simulink model "SchemaControlloDecentralizzatoSmartSixR2013a"  (Simulink 8.4)
settings: Solver=ode23  StartTime=0.0  StopTime=t(end)+Tf  FixedStep=T  RelTol=1e-3
PreLoadFcn:
  | initFunction
InitFcn:
  | initFunction
StopFcn:
  | figure
  | subplot(31,1)
  | plot(err_q.data(1:50))
  | subplot(312)
  | plot(err_dq.data(1:50))
  | subplot(313)
  | plot(err_ddq.data(1:50))
values from neighbouring files (symbols this model uses):
  FM = Kr^-1*Fv*Kr^-1    [ControlloreUnico.m]    (also in SimulazioneLsim.m = Kr^-1*Fv_att*Kr^-1; initFunction.m; initFunctionIm.m)
  Im = Kr^-1*Bconst*Kr^-1    [initFunction.m]    (also in initFunctionIm.m)
  KCA = diag([(-W(1,1)^2 + KM(1,1)*XR(1,1))/(KM(1,1)*KTA(1,1)*W(1,1)^2),             (-W(2,2)^2 + KM(2,2)*XR(2,2))/(KM(2,2)*KTA(2,2)*W(2,2)^2),             (-W(3,3)^2 + KM(3,3)*XR(3,3))/(KM(3,3)*KTA(3,3)*W(3,3)^2),             (-W(4,4)^2 + KM(4,4)*XR(4,4))/(KM(4,4)*KTA(4,4)*W(4,4)^2),             (-W(5,5)^2 + KM(5,5)*XR(5,5))/(KM(5,5)*KTA(5,5)*W(5,5)^2),             (-W(6,6)^2 + KM(6,6)*XR(6,6))/(KM(6,6)* ...(+20 chars)    [DesignControllersAcceleration_6.m]    (also in DesignControllersAcceleration_7.m; DiscreteControllersAcceleration_7.m)
  KCP = diag([(KTV(1,1)*W(1,1))/(2*KTP(1,1)*Z(1,1)),             (KTV(2,2)*W(2,2))/(2*KTP(2,2)*Z(2,2)),             (KTV(3,3)*W(3,3))/(2*KTP(3,3)*Z(3,3)),             (KTV(4,4)*W(4,4))/(2*KTP(4,4)*Z(4,4)),             (KTV(5,5)*W(5,5))/(2*KTP(5,5)*Z(5,5)),             (KTV(6,6)*W(6,6))/(2*KTP(6,6)*Z(6,6))])    [DesignControllersAcceleration_6.m]    (also in DesignControllersAcceleration_7.m; DesignControllersVelocity_6.m; DiscreteControllersAcceleration_7.m; DiscreteDesignControllersVelocity_6.m)
  KCV = diag([(2*KM(1,1)*KTA(1,1)*W(1,1)*XR(1,1)*Z(1,1))/(KTV(1,1)*(-W(1,1)^2 + KM(1,1)*XR(1,1))),             (2*KM(2,2)*KTA(2,2)*W(2,2)*XR(2,2)*Z(2,2))/(KTV(2,2)*(-W(2,2)^2 + KM(2,2)*XR(2,2))),             (2*KM(3,3)*KTA(3,3)*W(3,3)*XR(3,3)*Z(3,3))/(KTV(3,3)*(-W(3,3)^2 + KM(3,3)*XR(3,3))),             (2*KM(4,4)*KTA(4,4)*W(4,4)*XR(4,4)*Z(4,4))/(KTV(4,4)*(-W(4,4)^2 + KM(4,4)*XR(4,4))),             (2*KM( ...(+176 chars)    [DesignControllersAcceleration_6.m]    (also in DesignControllersAcceleration_7.m; DesignControllersVelocity_6.m = diag([(2*W(1,1)*Z(1,1))/(KM(1,1)*KTV(1,1)),             (2*W; DiscreteControllersAcceleration_7.m = diag([(rlkcv(1)*KM(1,1)*KTA(1,1)*W(1,1)*XR(1,1)*Z(1,1))/(KTV; DiscreteDesignControllersVelocity_6.m = diag([rlkcv(1)*(2*W(1,1)*Z(1,1))/(KM(1,1)*KTV(1,1)),        )
  KM = Kv^-1    [DesignControllersAcceleration_6.m]    (also in DesignControllersAcceleration_7.m; DesignControllersVelocity_6.m; DiscreteControllersAcceleration_7.m; DiscreteDesignControllersVelocity_6.m)
  KTA = diag([100 1 1 1 1 1])    [DesignControllersAcceleration_6.m]    (also in DesignControllersAcceleration_7.m = diag([1 1 1 1 1 1]); DiscreteControllersAcceleration_7.m = diag([1 1 1 1 1 1]))
  KTP = diag([9 1 1 1 1 1])    [DesignControllersAcceleration_6.m]    (also in DesignControllersAcceleration_7.m = diag([1 1 1 1 1 1]); DesignControllersVelocity_6.m = diag([1 1 1 1 1 1]); DiscreteControllersAcceleration_7.m = diag([1 1 1 1 1 1]); DiscreteDesignControllersVelocity_6.m = diag([1 1 1 1 1 1]))
  KTV = diag([4 1 1 1 1 1])    [DesignControllersAcceleration_6.m]    (also in DesignControllersAcceleration_7.m = diag([1 1 1 1 1 1]); DesignControllersVelocity_6.m = diag([1 1 1 1 1 1]); DiscreteControllersAcceleration_7.m = diag([1 1 1 1 1 1]); DiscreteDesignControllersVelocity_6.m = diag([1 1 1 1 1 1]))
  q0 = q0'    [initFunction.m]    (also in initFunctionIm.m)
  T = 0.05    [ComputeBconst_4.m]    (also in ControlloreUnico.m = 0.002; Identificazione_2.m = 0:1/F:(size(min_value,2)-1)*interval; Simulazione.m = 0.002; SimulazioneLsim.m = 0.002)
  TCA = diag([Tm(1,1) Tm(2,2) Tm(3,3) Tm(4,4) Tm(5,5) Tm(6,6)])    [DesignControllersAcceleration_6.m]    (also in DesignControllersAcceleration_7.m = diag([TM(1,1) TM(2,2) TM(3,3) TM(4,4) TM(5,5) TM(6,6)]); DiscreteControllersAcceleration_7.m = diag([TM(1,1) TM(2,2) TM(3,3) TM(4,4) TM(5,5) TM(6,6)]))
undefined symbols (not defined in the file or in its folder): Kr, Kt, Kv, La, Ra
libraries: simulink x18
(part 2 of 2)

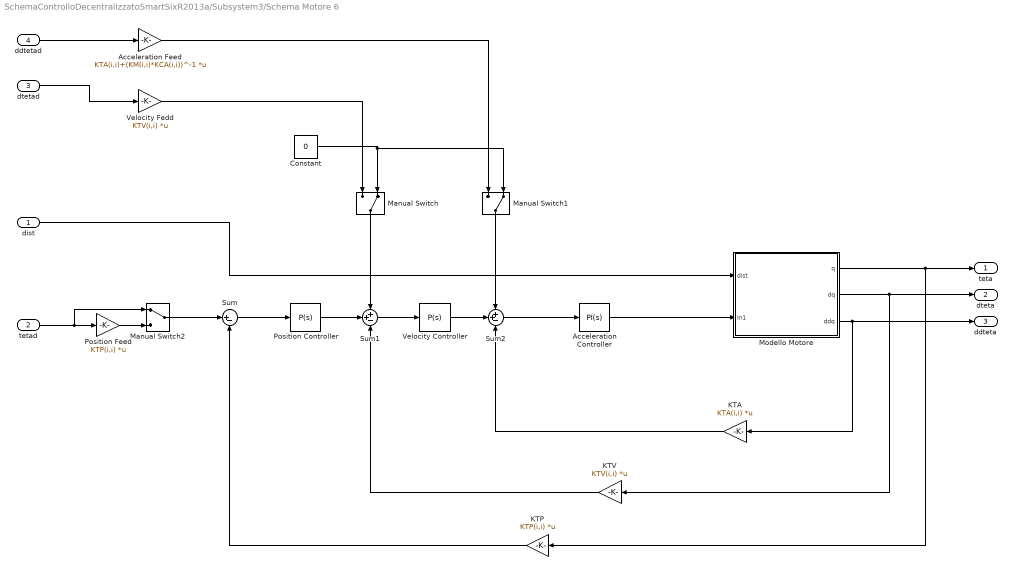
== system SchemaControlloDecentralizzatoSmartSixR2013a/Subsystem3/Schema Motore 6 ==
  dist : Inport  PortDimensions=1
  tetad : Inport  Port=2  PortDimensions=1
  dtetad : Inport  Port=3  PortDimensions=1
  ddtetad : Inport  Port=4  PortDimensions=1
  Acceleration Controller : simulink/Continuous/PID Controller  Controller=PI  TimeDomain=Continuous-time  SampleTime=-1  IntegratorMethod=Forward Euler  FilterMethod=Forward Euler  Form=Parallel  P=TCA(i,i)*KCA(i,i)  I=KCA(i,i)  D=0  N=100  InitialConditionSource=internal  InitialConditionForIntegrator=0  InitialConditionForFilter=0  ExternalReset=none  LimitOutput=off  UpperSaturationLimit=inf  LowerSaturationLimit=-inf  LinearizeAsGain=on  AntiWindupMode=none  Kb=1  TrackingMode=off  Kt=1  PParamMin=[]  PParamMax=[]  IParamMin=[]  IParamMax=[]  DParamMin=[]  DParamMax=[]  NParamMin=[]  NParamMax=[]  KbParamMin=[]  KbParamMax=[]  KtParamMin=[]  KtParamMax=[]  POutMin=[]  POutMax=[]  IOutMin=[]  IOutMax=[]  DOutMin=[]  DOutMax=[]  NOutMin=[]  NOutMax=[]  KbOutMin=[]  KbOutMax=[]  KtOutMin=[]  KtOutMax=[]  IntegratorOutMin=[]  IntegratorOutMax=[]  FilterOutMin=[]  FilterOutMax=[]  SumOutMin=[]  SumOutMax=[]  SumI1OutMin=[]  SumI1OutMax=[]  SumI2OutMin=[]  SumI2OutMax=[]  SumI3OutMin=[]  SumI3OutMax=[]  SumDOutMin=[]  SumDOutMax=[]  SaturationOutMin=[]  SaturationOutMax=[]  IntegratorContinuousStateAttributes=''  IntegratorStateMustResolveToSignalObject=off  IntegratorRTWStateStorageClass=Auto  FilterContinuousStateAttributes=''  FilterStateMustResolveToSignalObject=off  FilterRTWStateStorageClass=Auto  DifferentiatorICPrevScaledInput=0  DifferentiatorOutMin=[]  DifferentiatorOutMax=[]  UseFilter=on
  Acceleration Feed : Gain  Gain=KTA(i,i)+(KM(i,i)*KCA(i,i))^-1  Multiplication=Matrix(K*u)
  Constant : Constant  Value=0
  KTA : Gain  Gain=KTA(i,i)  Multiplication=Matrix(K*u)
  KTP : Gain  Gain=KTP(i,i)  Multiplication=Matrix(K*u)
  KTV : Gain  Gain=KTV(i,i)  Multiplication=Matrix(K*u)
  Manual Switch : ManualSwitch  CurrentSetting=0
  Manual Switch1 : ManualSwitch  CurrentSetting=0
  Manual Switch2 : ManualSwitch
  Modello Motore : Subsystem
  Position Controller : simulink/Continuous/PID Controller  Controller=P  TimeDomain=Continuous-time  SampleTime=-1  IntegratorMethod=Forward Euler  FilterMethod=Forward Euler  Form=Parallel  P=KCP(i,i)  I=1  D=0  N=100  InitialConditionSource=internal  InitialConditionForIntegrator=0  InitialConditionForFilter=0  ExternalReset=none  LimitOutput=off  UpperSaturationLimit=inf  LowerSaturationLimit=-inf  LinearizeAsGain=on  AntiWindupMode=none  Kb=1  TrackingMode=off  Kt=1  PParamMin=[]  PParamMax=[]  IParamMin=[]  IParamMax=[]  DParamMin=[]  DParamMax=[]  NParamMin=[]  NParamMax=[]  KbParamMin=[]  KbParamMax=[]  KtParamMin=[]  KtParamMax=[]  POutMin=[]  POutMax=[]  IOutMin=[]  IOutMax=[]  DOutMin=[]  DOutMax=[]  NOutMin=[]  NOutMax=[]  KbOutMin=[]  KbOutMax=[]  KtOutMin=[]  KtOutMax=[]  IntegratorOutMin=[]  IntegratorOutMax=[]  FilterOutMin=[]  FilterOutMax=[]  SumOutMin=[]  SumOutMax=[]  SumI1OutMin=[]  SumI1OutMax=[]  SumI2OutMin=[]  SumI2OutMax=[]  SumI3OutMin=[]  SumI3OutMax=[]  SumDOutMin=[]  SumDOutMax=[]  SaturationOutMin=[]  SaturationOutMax=[]  IntegratorContinuousStateAttributes=''  IntegratorStateMustResolveToSignalObject=off  IntegratorRTWStateStorageClass=Auto  FilterContinuousStateAttributes=''  FilterStateMustResolveToSignalObject=off  FilterRTWStateStorageClass=Auto  DifferentiatorICPrevScaledInput=0  DifferentiatorOutMin=[]  DifferentiatorOutMax=[]  UseFilter=on
  Position Feed : Gain  Gain=KTP(i,i)  Multiplication=Matrix(K*u)
  Sum : Sum  Inputs=|+-
  Sum1 : Sum  Inputs=++-
  Sum2 : Sum  Inputs=++-
  Velocity Controller : simulink/Continuous/PID Controller  Controller=P  TimeDomain=Continuous-time  SampleTime=-1  IntegratorMethod=Forward Euler  FilterMethod=Forward Euler  Form=Parallel  P=KCV(i,i)  I=1  D=0  N=100  InitialConditionSource=internal  InitialConditionForIntegrator=0  InitialConditionForFilter=0  ExternalReset=none  LimitOutput=off  UpperSaturationLimit=inf  LowerSaturationLimit=-inf  LinearizeAsGain=on  AntiWindupMode=none  Kb=1  TrackingMode=off  Kt=1  PParamMin=[]  PParamMax=[]  IParamMin=[]  IParamMax=[]  DParamMin=[]  DParamMax=[]  NParamMin=[]  NParamMax=[]  KbParamMin=[]  KbParamMax=[]  KtParamMin=[]  KtParamMax=[]  POutMin=[]  POutMax=[]  IOutMin=[]  IOutMax=[]  DOutMin=[]  DOutMax=[]  NOutMin=[]  NOutMax=[]  KbOutMin=[]  KbOutMax=[]  KtOutMin=[]  KtOutMax=[]  IntegratorOutMin=[]  IntegratorOutMax=[]  FilterOutMin=[]  FilterOutMax=[]  SumOutMin=[]  SumOutMax=[]  SumI1OutMin=[]  SumI1OutMax=[]  SumI2OutMin=[]  SumI2OutMax=[]  SumI3OutMin=[]  SumI3OutMax=[]  SumDOutMin=[]  SumDOutMax=[]  SaturationOutMin=[]  SaturationOutMax=[]  IntegratorContinuousStateAttributes=''  IntegratorStateMustResolveToSignalObject=off  IntegratorRTWStateStorageClass=Auto  FilterContinuousStateAttributes=''  FilterStateMustResolveToSignalObject=off  FilterRTWStateStorageClass=Auto  DifferentiatorICPrevScaledInput=0  DifferentiatorOutMin=[]  DifferentiatorOutMax=[]  UseFilter=on
  Velocity Fedd : Gain  Gain=KTV(i,i)  Multiplication=Matrix(K*u)
  teta : Outport  PortDimensions=1
  dteta : Outport  Port=2  PortDimensions=1
  ddteta : Outport  Port=3  PortDimensions=1
  wires:
  Sum/1 -> Position Controller/1
  Sum1/1 -> Velocity Controller/1
  Sum2/1 -> Acceleration Controller/1
  ddtetad/1 -> Acceleration Feed/1
  KTP/1 -> Sum/2
  Acceleration Controller/1 -> Modello Motore/2(In1)
  dist/1 -> Modello Motore/1(dist)
  Modello Motore/2(dq) -> dteta/1, KTV/1
  Modello Motore/1(q) -> teta/1, KTP/1
  Modello Motore/3(ddq) -> ddteta/1, KTA/1
  Position Controller/1 -> Sum1/2
  KTV/1 -> Sum1/3
  Manual Switch/1 -> Sum1/1
  KTA/1 -> Sum2/3
  Velocity Controller/1 -> Sum2/2
  Constant/1 -> Manual Switch1/2, Manual Switch/2
  Manual Switch1/1 -> Sum2/1
  tetad/1 -> Position Feed/1, Manual Switch2/1
  Manual Switch2/1 -> Sum/1
  Position Feed/1 -> Manual Switch2/2
  Velocity Fedd/1 -> Manual Switch/1
  Acceleration Feed/1 -> Manual Switch1/1
  dtetad/1 -> Velocity Fedd/1

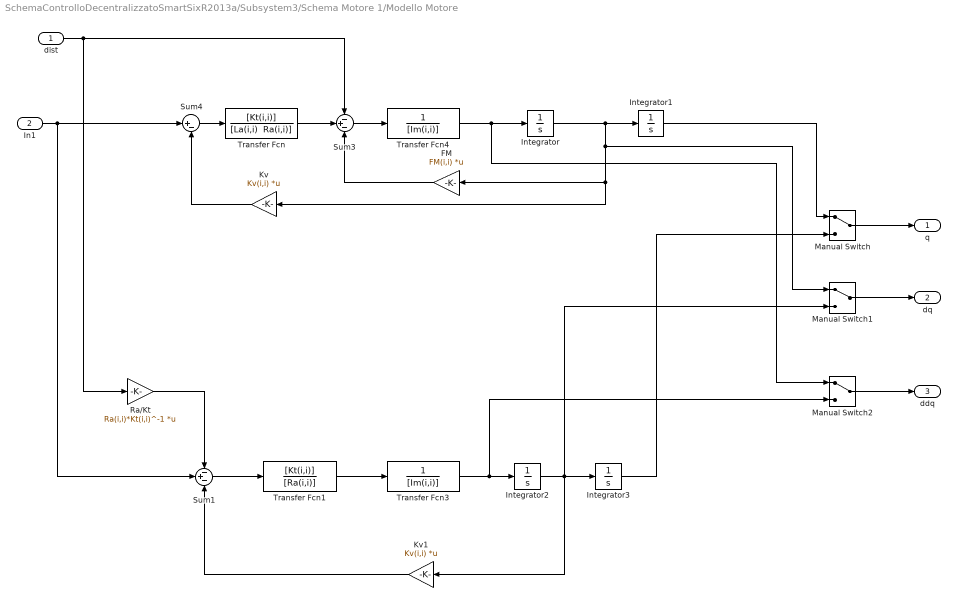
== system SchemaControlloDecentralizzatoSmartSixR2013a/Subsystem3/Schema Motore 1/Modello Motore ==
  dist : Inport
  In1 : Inport  Port=2
  FM : Gain  Gain=FM(i,i)  Multiplication=Matrix(K*u)
  Integrator : Integrator
  Integrator1 : Integrator  InitialCondition=q0(i)
  Integrator2 : Integrator
  Integrator3 : Integrator  InitialCondition=q0(i)
  Kv : Gain  Gain=Kv(i,i)  Multiplication=Matrix(K*u)
  Kv1 : Gain  Gain=Kv(i,i)  Multiplication=Matrix(K*u)
  Manual Switch : ManualSwitch
  Manual Switch1 : ManualSwitch
  Manual Switch2 : ManualSwitch
  Ra/Kt : Gain  Gain=Ra(i,i)*Kt(i,i)^-1  Multiplication=Matrix(K*u)
  Sum1 : Sum  Inputs=-+-
  Sum3 : Sum  Inputs=-+-
  Sum4 : Sum  Inputs=|+-
  Transfer Fcn : TransferFcn  Numerator=[Kt(i,i)]  Denominator="[La(i,i)  Ra(i,i)]"
  Transfer Fcn1 : TransferFcn  Numerator=[Kt(i,i)]  Denominator=[Ra(i,i)]
  Transfer Fcn3 : TransferFcn  Denominator=[Im(i,i)]
  Transfer Fcn4 : TransferFcn  Denominator=[Im(i,i)]
  q : Outport
  dq : Outport  Port=2
  ddq : Outport  Port=3
  wires:
  Manual Switch2/1 -> ddq/1
  Manual Switch1/1 -> dq/1
  Manual Switch/1 -> q/1
  Integrator/1 -> Kv/1, FM/1, Manual Switch1/1, Integrator1/1
  Kv/1 -> Sum4/2
  In1/1 -> Sum1/2, Sum4/1
  Sum4/1 -> Transfer Fcn/1
  Transfer Fcn/1 -> Sum3/2
  FM/1 -> Sum3/3
  Integrator1/1 -> Manual Switch/1
  dist/1 -> Ra/Kt/1, Sum3/1
  Ra/Kt/1 -> Sum1/1
  Sum1/1 -> Transfer Fcn1/1
  Transfer Fcn1/1 -> Transfer Fcn3/1
  Transfer Fcn3/1 -> Manual Switch2/2, Integrator2/1
  Integrator2/1 -> Manual Switch1/2, Kv1/1, Integrator3/1
  Kv1/1 -> Sum1/3
  Integrator3/1 -> Manual Switch/2
  Sum3/1 -> Transfer Fcn4/1
  Transfer Fcn4/1 -> Manual Switch2/1, Integrator/1

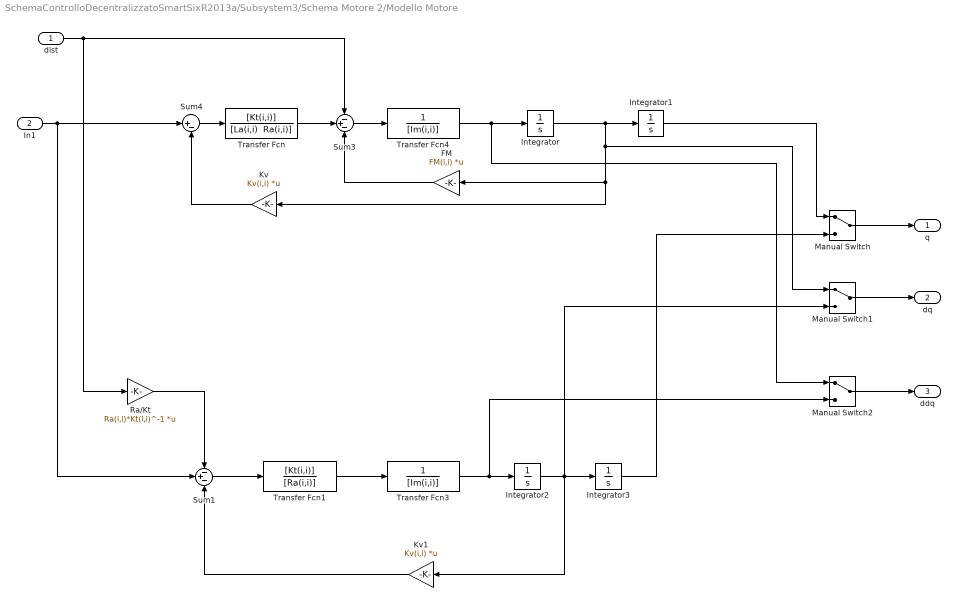
== system SchemaControlloDecentralizzatoSmartSixR2013a/Subsystem3/Schema Motore 2/Modello Motore ==
  dist : Inport
  In1 : Inport  Port=2
  FM : Gain  Gain=FM(i,i)  Multiplication=Matrix(K*u)
  Integrator : Integrator
  Integrator1 : Integrator  InitialCondition=q0(i)
  Integrator2 : Integrator
  Integrator3 : Integrator  InitialCondition=q0(i)
  Kv : Gain  Gain=Kv(i,i)  Multiplication=Matrix(K*u)
  Kv1 : Gain  Gain=Kv(i,i)  Multiplication=Matrix(K*u)
  Manual Switch : ManualSwitch
  Manual Switch1 : ManualSwitch
  Manual Switch2 : ManualSwitch
  Ra/Kt : Gain  Gain=Ra(i,i)*Kt(i,i)^-1  Multiplication=Matrix(K*u)
  Sum1 : Sum  Inputs=-+-
  Sum3 : Sum  Inputs=-+-
  Sum4 : Sum  Inputs=|+-
  Transfer Fcn : TransferFcn  Numerator=[Kt(i,i)]  Denominator="[La(i,i)  Ra(i,i)]"
  Transfer Fcn1 : TransferFcn  Numerator=[Kt(i,i)]  Denominator=[Ra(i,i)]
  Transfer Fcn3 : TransferFcn  Denominator=[Im(i,i)]
  Transfer Fcn4 : TransferFcn  Denominator=[Im(i,i)]
  q : Outport
  dq : Outport  Port=2
  ddq : Outport  Port=3
  wires:
  Manual Switch2/1 -> ddq/1
  Manual Switch1/1 -> dq/1
  Manual Switch/1 -> q/1
  Integrator/1 -> Kv/1, FM/1, Manual Switch1/1, Integrator1/1
  Kv/1 -> Sum4/2
  In1/1 -> Sum1/2, Sum4/1
  Sum4/1 -> Transfer Fcn/1
  Transfer Fcn/1 -> Sum3/2
  FM/1 -> Sum3/3
  Integrator1/1 -> Manual Switch/1
  dist/1 -> Ra/Kt/1, Sum3/1
  Ra/Kt/1 -> Sum1/1
  Sum1/1 -> Transfer Fcn1/1
  Transfer Fcn1/1 -> Transfer Fcn3/1
  Transfer Fcn3/1 -> Manual Switch2/2, Integrator2/1
  Integrator2/1 -> Manual Switch1/2, Kv1/1, Integrator3/1
  Kv1/1 -> Sum1/3
  Integrator3/1 -> Manual Switch/2
  Sum3/1 -> Transfer Fcn4/1
  Transfer Fcn4/1 -> Manual Switch2/1, Integrator/1

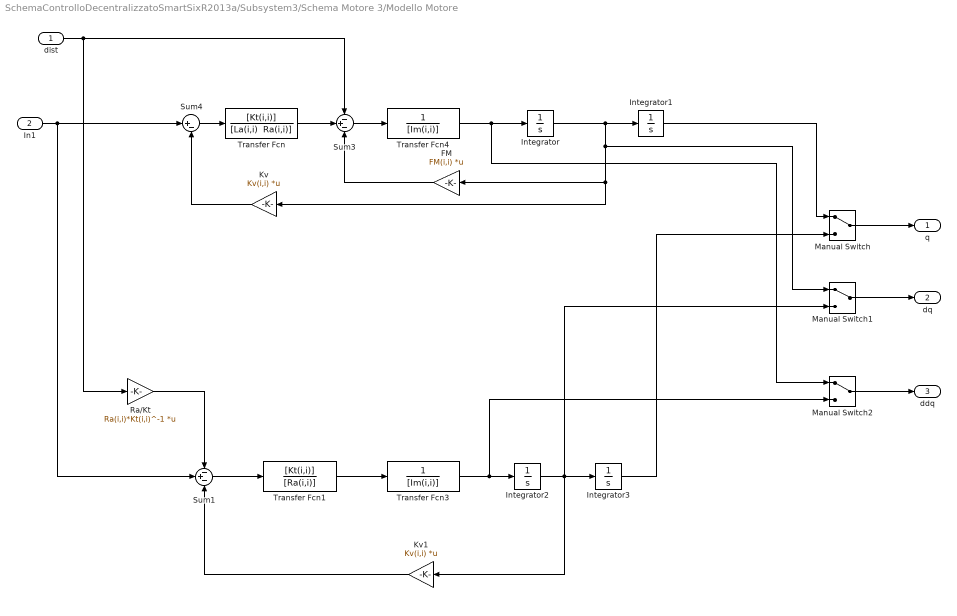
== system SchemaControlloDecentralizzatoSmartSixR2013a/Subsystem3/Schema Motore 3/Modello Motore ==
  dist : Inport
  In1 : Inport  Port=2
  FM : Gain  Gain=FM(i,i)  Multiplication=Matrix(K*u)
  Integrator : Integrator
  Integrator1 : Integrator  InitialCondition=q0(i)
  Integrator2 : Integrator
  Integrator3 : Integrator  InitialCondition=q0(i)
  Kv : Gain  Gain=Kv(i,i)  Multiplication=Matrix(K*u)
  Kv1 : Gain  Gain=Kv(i,i)  Multiplication=Matrix(K*u)
  Manual Switch : ManualSwitch
  Manual Switch1 : ManualSwitch
  Manual Switch2 : ManualSwitch
  Ra/Kt : Gain  Gain=Ra(i,i)*Kt(i,i)^-1  Multiplication=Matrix(K*u)
  Sum1 : Sum  Inputs=-+-
  Sum3 : Sum  Inputs=-+-
  Sum4 : Sum  Inputs=|+-
  Transfer Fcn : TransferFcn  Numerator=[Kt(i,i)]  Denominator="[La(i,i)  Ra(i,i)]"
  Transfer Fcn1 : TransferFcn  Numerator=[Kt(i,i)]  Denominator=[Ra(i,i)]
  Transfer Fcn3 : TransferFcn  Denominator=[Im(i,i)]
  Transfer Fcn4 : TransferFcn  Denominator=[Im(i,i)]
  q : Outport
  dq : Outport  Port=2
  ddq : Outport  Port=3
  wires:
  Manual Switch2/1 -> ddq/1
  Manual Switch1/1 -> dq/1
  Manual Switch/1 -> q/1
  Integrator/1 -> Kv/1, FM/1, Manual Switch1/1, Integrator1/1
  Kv/1 -> Sum4/2
  In1/1 -> Sum1/2, Sum4/1
  Sum4/1 -> Transfer Fcn/1
  Transfer Fcn/1 -> Sum3/2
  FM/1 -> Sum3/3
  Integrator1/1 -> Manual Switch/1
  dist/1 -> Ra/Kt/1, Sum3/1
  Ra/Kt/1 -> Sum1/1
  Sum1/1 -> Transfer Fcn1/1
  Transfer Fcn1/1 -> Transfer Fcn3/1
  Transfer Fcn3/1 -> Manual Switch2/2, Integrator2/1
  Integrator2/1 -> Manual Switch1/2, Kv1/1, Integrator3/1
  Kv1/1 -> Sum1/3
  Integrator3/1 -> Manual Switch/2
  Sum3/1 -> Transfer Fcn4/1
  Transfer Fcn4/1 -> Manual Switch2/1, Integrator/1

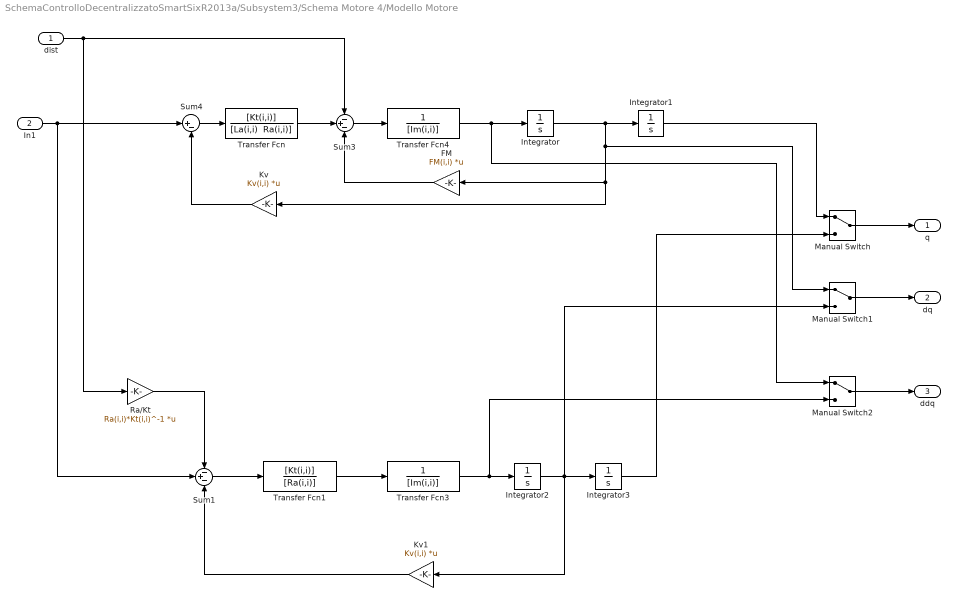
== system SchemaControlloDecentralizzatoSmartSixR2013a/Subsystem3/Schema Motore 4/Modello Motore ==
  dist : Inport
  In1 : Inport  Port=2
  FM : Gain  Gain=FM(i,i)  Multiplication=Matrix(K*u)
  Integrator : Integrator
  Integrator1 : Integrator  InitialCondition=q0(i)
  Integrator2 : Integrator
  Integrator3 : Integrator  InitialCondition=q0(i)
  Kv : Gain  Gain=Kv(i,i)  Multiplication=Matrix(K*u)
  Kv1 : Gain  Gain=Kv(i,i)  Multiplication=Matrix(K*u)
  Manual Switch : ManualSwitch
  Manual Switch1 : ManualSwitch
  Manual Switch2 : ManualSwitch
  Ra/Kt : Gain  Gain=Ra(i,i)*Kt(i,i)^-1  Multiplication=Matrix(K*u)
  Sum1 : Sum  Inputs=-+-
  Sum3 : Sum  Inputs=-+-
  Sum4 : Sum  Inputs=|+-
  Transfer Fcn : TransferFcn  Numerator=[Kt(i,i)]  Denominator="[La(i,i)  Ra(i,i)]"
  Transfer Fcn1 : TransferFcn  Numerator=[Kt(i,i)]  Denominator=[Ra(i,i)]
  Transfer Fcn3 : TransferFcn  Denominator=[Im(i,i)]
  Transfer Fcn4 : TransferFcn  Denominator=[Im(i,i)]
  q : Outport
  dq : Outport  Port=2
  ddq : Outport  Port=3
  wires:
  Manual Switch2/1 -> ddq/1
  Manual Switch1/1 -> dq/1
  Manual Switch/1 -> q/1
  Integrator/1 -> Kv/1, FM/1, Manual Switch1/1, Integrator1/1
  Kv/1 -> Sum4/2
  In1/1 -> Sum1/2, Sum4/1
  Sum4/1 -> Transfer Fcn/1
  Transfer Fcn/1 -> Sum3/2
  FM/1 -> Sum3/3
  Integrator1/1 -> Manual Switch/1
  dist/1 -> Ra/Kt/1, Sum3/1
  Ra/Kt/1 -> Sum1/1
  Sum1/1 -> Transfer Fcn1/1
  Transfer Fcn1/1 -> Transfer Fcn3/1
  Transfer Fcn3/1 -> Manual Switch2/2, Integrator2/1
  Integrator2/1 -> Manual Switch1/2, Kv1/1, Integrator3/1
  Kv1/1 -> Sum1/3
  Integrator3/1 -> Manual Switch/2
  Sum3/1 -> Transfer Fcn4/1
  Transfer Fcn4/1 -> Manual Switch2/1, Integrator/1

== system SchemaControlloDecentralizzatoSmartSixR2013a/Subsystem3/Schema Motore 5/Modello Motore ==
  dist : Inport
  In1 : Inport  Port=2
  FM : Gain  Gain=FM(i,i)  Multiplication=Matrix(K*u)
  Integrator : Integrator
  Integrator1 : Integrator  InitialCondition=q0(i)
  Integrator2 : Integrator
  Integrator3 : Integrator  InitialCondition=q0(i)
  Kv : Gain  Gain=Kv(i,i)  Multiplication=Matrix(K*u)
  Kv1 : Gain  Gain=Kv(i,i)  Multiplication=Matrix(K*u)
  Manual Switch : ManualSwitch
  Manual Switch1 : ManualSwitch
  Manual Switch2 : ManualSwitch
  Ra/Kt : Gain  Gain=Ra(i,i)*Kt(i,i)^-1  Multiplication=Matrix(K*u)
  Sum1 : Sum  Inputs=-+-
  Sum3 : Sum  Inputs=-+-
  Sum4 : Sum  Inputs=|+-
  Transfer Fcn : TransferFcn  Numerator=[Kt(i,i)]  Denominator="[La(i,i)  Ra(i,i)]"
  Transfer Fcn1 : TransferFcn  Numerator=[Kt(i,i)]  Denominator=[Ra(i,i)]
  Transfer Fcn3 : TransferFcn  Denominator=[Im(i,i)]
  Transfer Fcn4 : TransferFcn  Denominator=[Im(i,i)]
  q : Outport
  dq : Outport  Port=2
  ddq : Outport  Port=3
  wires:
  Manual Switch2/1 -> ddq/1
  Manual Switch1/1 -> dq/1
  Manual Switch/1 -> q/1
  Integrator/1 -> Kv/1, FM/1, Manual Switch1/1, Integrator1/1
  Kv/1 -> Sum4/2
  In1/1 -> Sum1/2, Sum4/1
  Sum4/1 -> Transfer Fcn/1
  Transfer Fcn/1 -> Sum3/2
  FM/1 -> Sum3/3
  Integrator1/1 -> Manual Switch/1
  dist/1 -> Ra/Kt/1, Sum3/1
  Ra/Kt/1 -> Sum1/1
  Sum1/1 -> Transfer Fcn1/1
  Transfer Fcn1/1 -> Transfer Fcn3/1
  Transfer Fcn3/1 -> Manual Switch2/2, Integrator2/1
  Integrator2/1 -> Manual Switch1/2, Kv1/1, Integrator3/1
  Kv1/1 -> Sum1/3
  Integrator3/1 -> Manual Switch/2
  Sum3/1 -> Transfer Fcn4/1
  Transfer Fcn4/1 -> Manual Switch2/1, Integrator/1

== system SchemaControlloDecentralizzatoSmartSixR2013a/Subsystem3/Schema Motore 6/Modello Motore ==
  dist : Inport
  In1 : Inport  Port=2
  FM : Gain  Gain=FM(i,i)  Multiplication=Matrix(K*u)
  Integrator : Integrator
  Integrator1 : Integrator  InitialCondition=q0(i)
  Integrator2 : Integrator
  Integrator3 : Integrator  InitialCondition=q0(i)
  Kv : Gain  Gain=Kv(i,i)  Multiplication=Matrix(K*u)
  Kv1 : Gain  Gain=Kv(i,i)  Multiplication=Matrix(K*u)
  Manual Switch : ManualSwitch
  Manual Switch1 : ManualSwitch
  Manual Switch2 : ManualSwitch
  Ra/Kt : Gain  Gain=Ra(i,i)*Kt(i,i)^-1  Multiplication=Matrix(K*u)
  Sum1 : Sum  Inputs=-+-
  Sum3 : Sum  Inputs=-+-
  Sum4 : Sum  Inputs=|+-
  Transfer Fcn : TransferFcn  Numerator=[Kt(i,i)]  Denominator="[La(i,i)  Ra(i,i)]"
  Transfer Fcn1 : TransferFcn  Numerator=[Kt(i,i)]  Denominator=[Ra(i,i)]
  Transfer Fcn3 : TransferFcn  Denominator=[Im(i,i)]
  Transfer Fcn4 : TransferFcn  Denominator=[Im(i,i)]
  q : Outport
  dq : Outport  Port=2
  ddq : Outport  Port=3
  wires:
  Manual Switch2/1 -> ddq/1
  Manual Switch1/1 -> dq/1
  Manual Switch/1 -> q/1
  Integrator/1 -> Kv/1, FM/1, Manual Switch1/1, Integrator1/1
  Kv/1 -> Sum4/2
  In1/1 -> Sum1/2, Sum4/1
  Sum4/1 -> Transfer Fcn/1
  Transfer Fcn/1 -> Sum3/2
  FM/1 -> Sum3/3
  Integrator1/1 -> Manual Switch/1
  dist/1 -> Ra/Kt/1, Sum3/1
  Ra/Kt/1 -> Sum1/1
  Sum1/1 -> Transfer Fcn1/1
  Transfer Fcn1/1 -> Transfer Fcn3/1
  Transfer Fcn3/1 -> Manual Switch2/2, Integrator2/1
  Integrator2/1 -> Manual Switch1/2, Kv1/1, Integrator3/1
  Kv1/1 -> Sum1/3
  Integrator3/1 -> Manual Switch/2
  Sum3/1 -> Transfer Fcn4/1
  Transfer Fcn4/1 -> Manual Switch2/1, Integrator/1
